simulink model "fuzzyfis_withload"  (R2024b)
settings: Solver=ode45  StartTime=0  StopTime=30  MaxStep=0.2  RelTol=1e-3  AbsTol=1e-6
PreLoadFcn:
  | tank = readfis('tank');
libraries: fuzblock x1
CloseFcn:
  | AnimFigH = findobj(0,'Name', 'Tank Demo'); close(AnimFigH)
  | 
  | clear tank AnimFigH
settings Model: Creator=The MathWorks, Inc.  LastModifiedBy=ysemila07
settings SolverCC: AutoScaleAbsTol=off  AlgebraicLoopSolver=TrustRegion  MaxZcPerStep=1
settings DataIOCC: SaveFormat=Array  SaveOutput=off  SaveTime=off  ReturnWorkspaceOutputs=off
settings OptimizationCC: BlockReduction=off  BooleanDataType=off  ExpressionDepthLimit=2147483647  InitFltsAndDblsToZero=on  LifeSpan=inf
settings DebuggingCC: SaveWithParameterizedLinksMsg=none  UnderspecifiedInitializationDetection=Classic  MergeDetectMultiDrivingBlocksExec=none  SignalResolutionControl=TryResolveAllWithWarning  MultiTaskDSMMsg=warning  MultiTaskCondExecSysMsg=none  FcnCallInpInsideContextMsg=warning  UnconnectedInputMsg=warning  UnconnectedOutputMsg=warning  UnconnectedLineMsg=warning  StateNameClashWarn=warning  SFUnexpectedBacktrackingDiag=warning  SFNoUnconditionalDefaultTransitionDiag=warning  SFExecutionAtInitializationDiag=none  ArithmeticOperatorsInVariantConditions=warning
settings HardwareCC: ProdBitPerPointer=32  ProdBitPerSizeT=32  ProdBitPerPtrDiffT=32  ProdLargestAtomicFloat=None  ProdIntDivRoundTo=Undefined  ProdEndianess=Unspecified  ProdWordSize=32  ProdHWDeviceType=32-bit Generic  TargetUnknown=on
settings ModelReferenceCC: EnableRefExpFcnMdlSchedulingChecks=on  PropagateSignalLabelsOutOfModel=off
settings SFSimCC: SimUseLocalCustomCode=off  CustomCodeUndefinedFunction=UseInterfaceOnly
settings RTWCC: TemplateMakefile=grt_unix.tmf  RTWUseLocalCustomCode=off  GPUComputeCapability=3.5  DLArmComputeVersion=19.05
settings CodeAppCC: StateflowObjectComments=on
settings GRTTargetCC: TargetFcnLib=ansi_tfl_tmw.mat  TargetLangStandard=C89/C90 (ANSI)  CombineOutputUpdateFcns=off  GRTInterface=on
settings ConfigComp: CovMetricSettings=dw  CovSaveCumulativeToWorkspaceVar=on  CovSaveSingleToWorkspaceVar=on  CovExternalEMLEnable=off

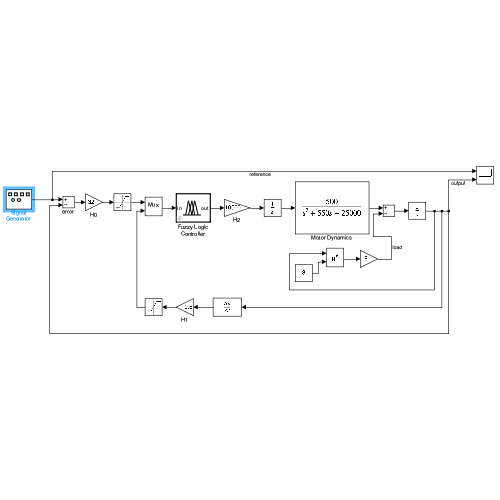
[thumbnail: Simulink's stored preview of the top-level diagram]
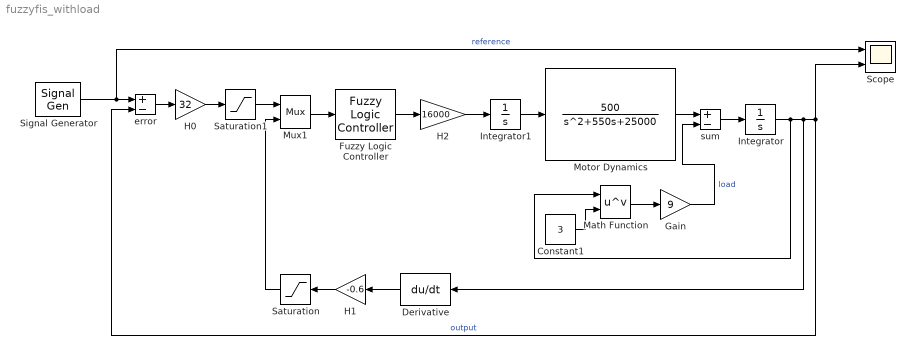
== system fuzzyfis_withload ==
  Constant1 : Constant  Value=3
  Derivative : Derivative
  Fuzzy Logic Controller : fuzblock/Fuzzy Logic  Controller  FIS=motor_control  OutputSampleNumber=101  DataType=double  FuzzifiedInputs=off  RuleFiringStrengths=off  RuleOutputs=off  AggregatedOutputs=off  SimulateUsing=Interpreted execution  OutOfRangeInputValueMessage=warning  NoRuleFiredMessage=warning  EmptyOutputFuzzySetMessage=warning
  Gain : Gain  Gain=9
  H0 : Gain  Gain=32
  H1 : Gain  Gain=-0.6
  H2 : Gain  Gain=16000
  Integrator : Integrator
  Integrator1 : Integrator
  Math Function : Math  Operator=pow
  Motor Dynamics : TransferFcn  Numerator=[500]  Denominator=[1 550 25000]
  Mux1 : Mux  Inputs=2
  Saturation : Saturate  UpperLimit=1  LowerLimit=-1
  Saturation1 : Saturate  UpperLimit=1  LowerLimit=-1
  Scope : Scope  NumInputPorts=2
  Signal Generator : SignalGenerator  WaveForm=square  Frequency=0.5  Units=rad/sec
  error : Sum  Inputs=+-  InputSameDT=on  SaturateOnIntegerOverflow=on  OutDataTypeStr=Inherit: Same as first input
  sum : Sum  Inputs=+-  InputSameDT=on  SaturateOnIntegerOverflow=on  OutDataTypeStr=Inherit: Same as first input
  wires:
  Mux1/1 -> Fuzzy Logic Controller/1
  Integrator/1 -> Derivative/1, Scope/2, error/2, Math Function/1  "output"
  Signal Generator/1 -> Scope/1, error/1  "reference"
  Fuzzy Logic Controller/1 -> H2/1
  error/1 -> H0/1
  H2/1 -> Integrator1/1
  Integrator1/1 -> Motor Dynamics/1
  H0/1 -> Saturation1/1
  Saturation1/1 -> Mux1/1
  Saturation/1 -> Mux1/2
  H1/1 -> Saturation/1
  Derivative/1 -> H1/1
  Math Function/1 -> Gain/1
  Constant1/1 -> Math Function/2
  sum/1 -> Integrator/1
  Motor Dynamics/1 -> sum/1
  Gain/1 -> sum/2  "load"
